simulink model "Pod_elev_plant_linear"  (R2022b)
settings: Solver=VariableStepAuto  StartTime=0.0  StopTime=10.0  RelTol=1e-3
undefined symbols (not defined in the file): fix_conseg, JLreg, JMreg, Kkeg, Kveg
libraries: slctrlblks x1
settings Model: Creator=ohadformanair  LastModifiedBy=ohadformanair

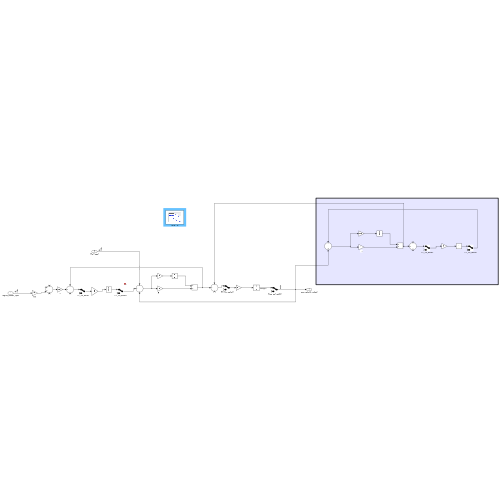
[thumbnail: Simulink's stored preview of the top-level diagram]
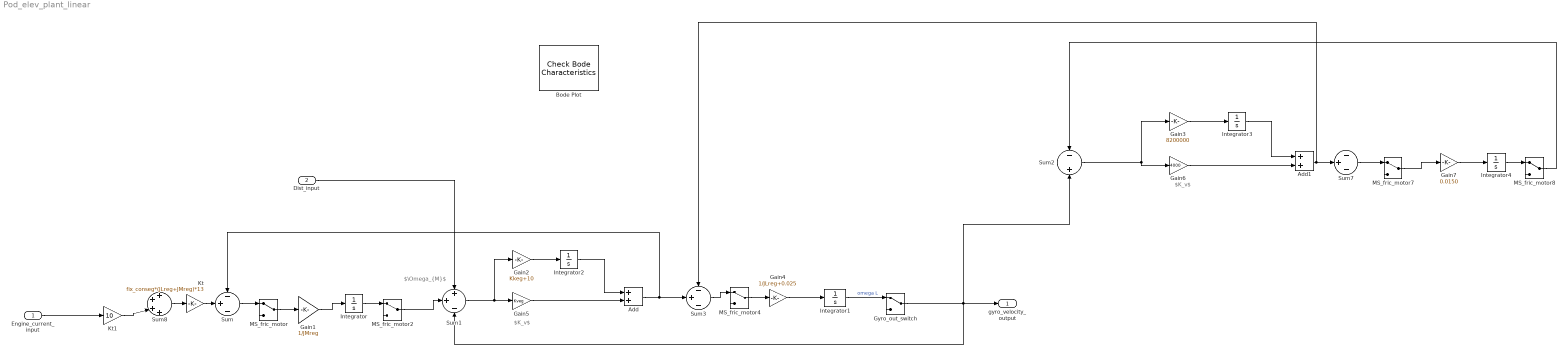
== system Pod_elev_plant_linear ==
  note: $K_v$
  note: $K_v$
  note: $\Omega_{M}$
  Engine_current_input : Inport
  Dist_input : Inport  Port=2
  Add : Sum
  Add1 : Sum
  Bode Plot : slctrlblks/Model Verification/Check Bode  Characteristics  InstantiateOnLoad=on  SaveOperatingPoints=off  LinearizationIOs={'/Dist_input', 1, 'in', 'off', '';'/Engine_current_input', 1, 'in', 'off', '';'/Gyro_out_switch', 1, 'out', 'off', ''}  LinearizeAt=SnapshotTimes  SnapshotTimes=[0]  TriggerType=rising  SampleTime=auto  RateConversionMethod=zoh  PreWarpFreq=10  UseExactDelayModel=off  UseFullBlockNameLabels=off  UseBusSignalLabels=off  enabled=on  stopWhenAssertionFail=off  export=off  ViewDlgPos=[62 219 1265 798]  OpenViewOnLoad=off  LaunchViewOnOpen=off  FrequencyUnits=Hz  MagnitudeUnits=dB  PhaseUnits=deg  TimeUnits=seconds  EnableUpperBound=off  UpperBoundFrequencies=[]  UpperBoundMagnitudes=[]  EnableLowerBound=off  LowerBoundFrequencies=[]  LowerBoundMagnitudes=[]
  Gain1 : Gain  Gain=1/JMreg
  Gain2 : Gain  Gain=Kkeg+10
  Gain3 : Gain  Gain=8200000
  Gain4 : Gain  Gain=1/JLreg+0.025
  Gain5 : Gain  Gain=Kveg
  Gain6 : Gain  Gain=4000
  Gain7 : Gain  Gain=0.0150
  Gyro_out_switch : ManualSwitch
  Integrator{,1..4} (5 alike) : Integrator
  Kt : Gain  Gain=fix_conseg*(JLreg+JMreg)*13
  Kt1 : Gain  Gain=10
  MS_fric_motor{,2,4,7..8} (5 alike) : ManualSwitch
  Sum : Sum  Inputs=-+-
  Sum1 : Sum  Inputs=++-
  Sum2 : Sum  Inputs=-+
  Sum3 : Sum  Inputs=-+-
  Sum7 : Sum  Inputs=-+-
  Sum8 : Sum  Inputs=++++
  gyro_velocity_output : Outport
  wires:
  Gain1/1 -> Integrator/1
  Sum1/1 -> Gain5/1, Gain2/1
  Integrator2/1 -> Add/1
  Kt1/1 -> Sum8/3
  Gain5/1 -> Add/2
  Gain6/1 -> Add1/2
  Gain7/1 -> Integrator4/1
  Add/1 -> Sum3/2, Sum/1
  Gain3/1 -> Integrator3/1
  Integrator3/1 -> Add1/1
  MS_fric_motor8/1 -> Sum2/1
  Gyro_out_switch/1 -> Sum2/2, Sum1/3, gyro_velocity_output/1
  MS_fric_motor2/1 -> Sum1/2
  Integrator4/1 -> MS_fric_motor8/1
  Sum7/1 -> MS_fric_motor7/1
  Gain2/1 -> Integrator2/1
  Sum8/1 -> Kt/1
  MS_fric_motor/1 -> Gain1/1
  Sum2/1 -> Gain6/1, Gain3/1
  Integrator1/1 -> Gyro_out_switch/1  "omega L"
  Engine_current_input/1 -> Kt1/1
  Integrator/1 -> MS_fric_motor2/1
  Sum3/1 -> MS_fric_motor4/1
  Gain4/1 -> Integrator1/1
  MS_fric_motor7/1 -> Gain7/1
  Kt/1 -> Sum/2
  MS_fric_motor4/1 -> Gain4/1
  Sum/1 -> MS_fric_motor/1
  Add1/1 -> Sum7/2, Sum3/1
  Dist_input/1 -> Sum1/1
